simulink model "ydxmpc2"  (R2022a)
settings: Solver=VariableStepAuto  StartTime=0.0  StopTime=50  RelTol=1e-3
values from neighbouring files (symbols this model uses):
  cx = 0:0.1:120    [mpcdlx_ref.m]
  cy = dy1/2.*(1+tanh(z1))-dy2/2.*(1+tanh(z2))    [mpcdlx_ref.m]
  r_k = abs(dd_y) ./ (1+d_y.^2).^(3/2)    [mpcdlx_ref.m]
  r_yaw = atan2(dif_yyyy , dif_xxxx)    [mpcdlx_ref.m]
libraries: Solver_SF x1, simulink x1
settings Model: Creator=wenju  LastModifiedBy=wenju

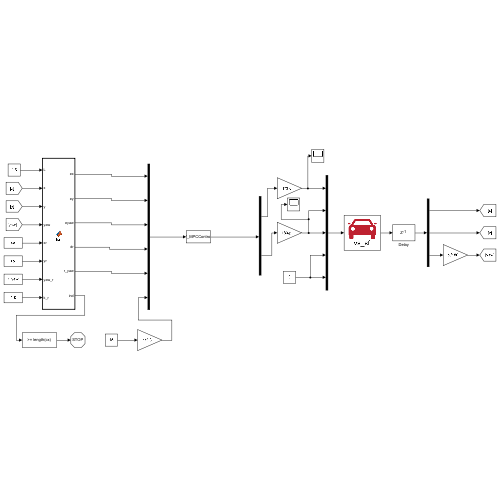
[thumbnail: Simulink's stored preview of the top-level diagram]
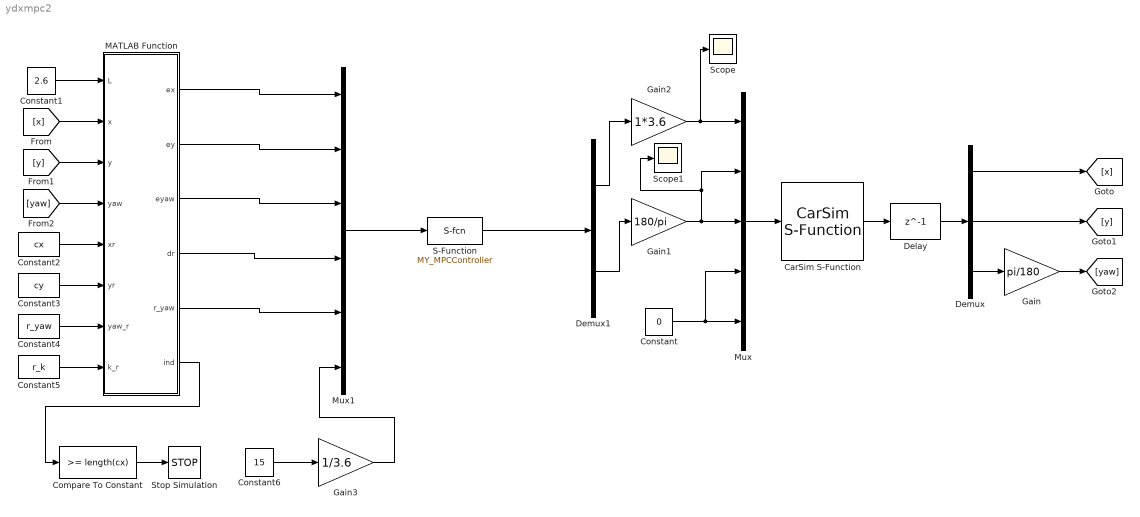
== system ydxmpc2 ==
  CarSim S-Function : Solver_SF/CarSim S-Function  Priority=1  SIMFILE=simfile.sim  Run_RTs=off  vs_state_ind=Run  StopMode_ind=Vehicle Model
  Compare To Constant : simulink/Logic and Bit Operations/Compare To Constant  relop=>=  const=length(cx)  OutDataTypeStr=boolean
  Constant : Constant  Value=0
  Constant1 : Constant  Value=2.6
  Constant2 : Constant  Value=cx
  Constant3 : Constant  Value=cy
  Constant4 : Constant  Value=r_yaw
  Constant5 : Constant  Value=r_k
  Constant6 : Constant  Value=15
  Delay : Delay  DelayLength=1  InitialCondition=0  UseCircularBuffer=on
  Demux : Demux  Outputs=3
  Demux1 : Demux  Outputs=2
  Gain : Gain  Gain=pi/180
  Gain1 : Gain  Gain=180/pi
  Gain2 : Gain  Gain=1*3.6
  Gain3 : Gain  Gain=1/3.6
  MATLAB Function : MATLAB Function  TreatAsAtomicUnit=on
  Mux : Mux  Inputs=5
  Mux1 : Mux  Inputs=6
  S-Function : S-Function  FunctionName=MY_MPCController  SFunctionDeploymentMode=off  EnableBusSupport=off
  Scope : Scope
  Scope1 : Scope
  Stop Simulation : Stop
  wires:
  CarSim S-Function/1 -> Delay/1
  Delay/1 -> Demux/1
  Demux/1 -> [x]
  Demux/2 -> [y]
  Demux/3 -> Gain/1
  Gain/1 -> [yaw]
  Mux/1 -> CarSim S-Function/1
  Constant/1 -> Mux/4, Mux/5
  Gain1/1 -> Scope1/1, Mux/2, Mux/3
  Gain2/1 -> Scope/1, Mux/1
  Constant1/1 -> MATLAB Function/1(L)
  [x] -> MATLAB Function/2(x)
  [y] -> MATLAB Function/3(y)
  [yaw] -> MATLAB Function/4(yaw)
  Constant2/1 -> MATLAB Function/5(xr)
  Constant3/1 -> MATLAB Function/6(yr)
  Constant5/1 -> MATLAB Function/8(k_r)
  Constant4/1 -> MATLAB Function/7(yaw_r)
  MATLAB Function/1(ex) -> Mux1/1
  MATLAB Function/2(ey) -> Mux1/2
  MATLAB Function/3(eyaw) -> Mux1/3
  MATLAB Function/4(dr) -> Mux1/4
  MATLAB Function/5(r_yaw) -> Mux1/5
  Constant6/1 -> Gain3/1
  Gain3/1 -> Mux1/6
  Demux1/1 -> Gain2/1
  Demux1/2 -> Gain1/1
  MATLAB Function/6(ind) -> Compare To Constant/1
  Compare To Constant/1 -> Stop Simulation/1
  Mux1/1 -> S-Function/1
  S-Function/1 -> Demux1/1

== matlab function ydxmpc2/MATLAB Function ==
  data: L input; ex output; x input; y input; yaw input; xr input; yr input; yaw_r input; k_r input; ey output; eyaw output; dr output; r_yaw output; ind output
function [ex,ey,eyaw,dr,r_yaw,ind] = fcn(L,x,y,yaw,xr,yr,yaw_r,k_r)
%1.寻找匹配点（车辆离期望路径最近的点）   
    n=length(xr);
    d_min=(x-xr(1))^2+(y-yr(1))^2;
    min=1;
    for i=1:n
        d=(x-xr(i))^2+(y-yr(i))^2;
        if d<d_min
            d_min=d;
            min=i;
        end
    end
    ind=min;

%2.计算3个误差状态[ex,ey,eyaw]
    ex=x-xr(ind);
    ey=y-yr(ind);

    eyaw=yaw-yaw_r(ind);

%3.计算计算参考前轮转角dr
    dr=atan(L*k_r(ind));

%4.参考航向角也输出  
    r_yaw=yaw_r(ind);

end
